simulink model "DC_MOTOR11"  (R2018a)
settings: Solver=FixedStepAuto  StartTime=0.0  StopTime=8  FixedStep=0.00001  RelTol=1e-3
values from neighbouring files (symbols this model uses):
  Bm = 0.0006    [dc1.m]
  Jm = 0.00233    [dc1.m]
  Kmm = 1    [dc1.m]
  Lam = 0.0017    [dc1.m]
  Lfm = 0.08    [dc1.m]
  Ram = 0.33    [dc1.m]
  Rfm = 3.33,    [dc1.m]
settings Model: ModifiedByFormat=LENOVO  Creator=Petar  LastModifiedBy=LENOVO

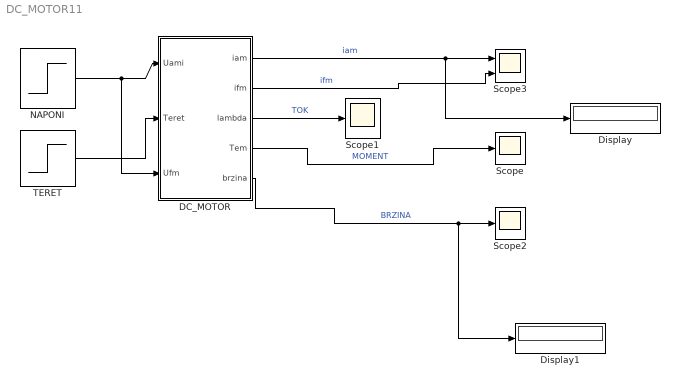
== system DC_MOTOR11 ==
  DC_MOTOR : Subsystem
  Display : Display
  Display1 : Display
  NAPONI : Step  After=24  SampleTime=0
  Scope : Scope
  Scope1 : Scope
  Scope2 : Scope
  Scope3 : Scope  NumInputPorts=2
  TERET : Step  After=27  SampleTime=0
  wires:
  NAPONI/1 -> DC_MOTOR/3(Ufm), DC_MOTOR/1("\tUami")
  TERET/1 -> DC_MOTOR/2(Teret)
  DC_MOTOR/1(iam) -> Display/1, Scope3/1  "iam"
  DC_MOTOR/2(ifm) -> Scope3/2  "ifm"
  DC_MOTOR/3(lambda) -> Scope1/1  "TOK"
  DC_MOTOR/4(Tem) -> Scope/1  "MOMENT"
  DC_MOTOR/5(brzina) -> Display1/1, Scope2/1  "BRZINA"

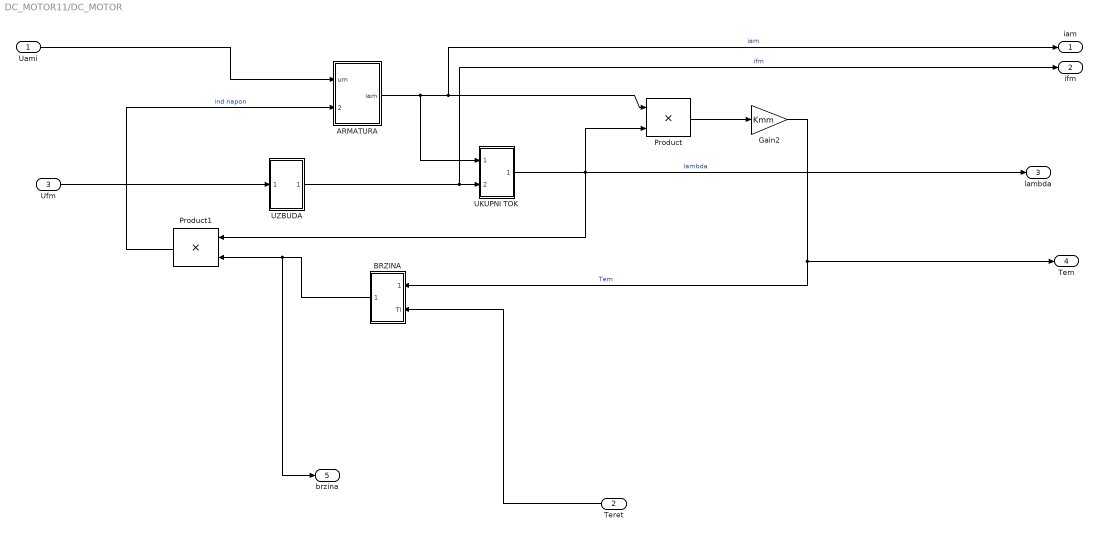
== system DC_MOTOR11/DC_MOTOR ==
  "\tUami" : Inport
  Teret : Inport  Port=2
  Ufm : Inport  Port=3
  ARMATURA : Subsystem
  BRZINA : Subsystem
  Gain2 : Gain  Gain=Kmm
  Product : Product
  Product1 : Product
  UKUPNI TOK : Subsystem
  UZBUDA : Subsystem
  iam : Outport
  ifm : Outport  Port=2
  lambda : Outport  Port=3
  Tem : Outport  Port=4
  brzina : Outport  Port=5
  wires:
  Gain2/1 -> Tem/1, BRZINA/1(Tem)  "Tem"
  UZBUDA/1(ifm) -> ifm/1, UKUPNI TOK/2(ifm)  "ifm"
  Teret/1 -> BRZINA/2(Tl)
  ARMATURA/1(iam) -> UKUPNI TOK/1(iam), iam/1, Product/1  "iam"
  BRZINA/1(wm) -> brzina/1, Product1/2
  Product1/1 -> ARMATURA/2(ind napon)  "ind napon"
  "\tUami"/1 -> ARMATURA/1(um)
  Product/1 -> Gain2/1
  UKUPNI TOK/1(lambda) -> lambda/1, Product1/1, Product/2  "lambda"
  Ufm/1 -> UZBUDA/1(Ufm)

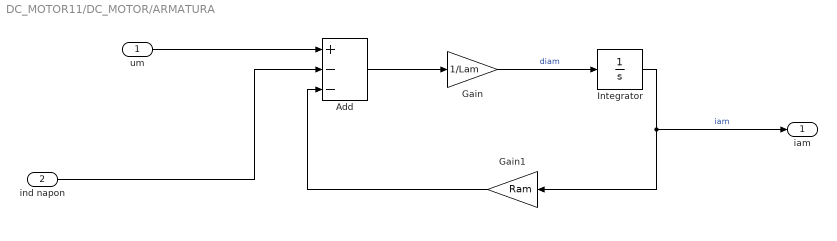
== system DC_MOTOR11/DC_MOTOR/ARMATURA ==
  um : Inport
  ind napon : Inport  Port=2
  Add : Sum  Inputs=+--
  Gain : Gain  Gain=1/Lam
  Gain1 : Gain  Gain=Ram
  Integrator : Integrator
  iam : Outport
  wires:
  Integrator/1 -> iam/1, Gain1/1  "iam"
  Gain/1 -> Integrator/1  "diam"
  Gain1/1 -> Add/3
  um/1 -> Add/1
  Add/1 -> Gain/1
  ind napon/1 -> Add/2

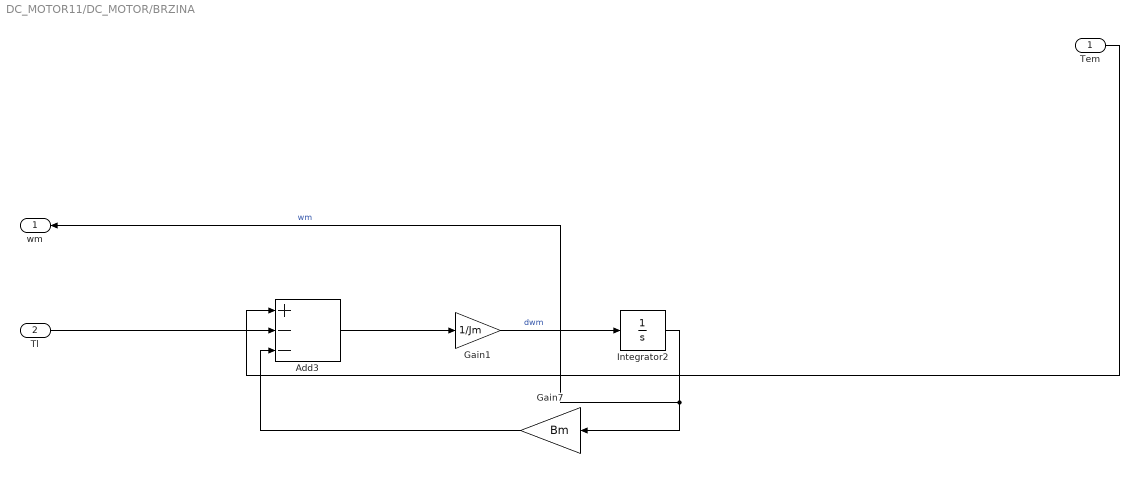
== system DC_MOTOR11/DC_MOTOR/BRZINA ==
  Tem : Inport
  Tl : Inport  Port=2
  Add3 : Sum  Inputs=+--
  Gain1 : Gain  Gain=1/Jm
  Gain7 : Gain  Gain=Bm
  Integrator2 : Integrator
  wm : Outport
  wires:
  Gain1/1 -> Integrator2/1  "dwm"
  Tl/1 -> Add3/2
  Gain7/1 -> Add3/3
  Integrator2/1 -> wm/1, Gain7/1  "wm"
  Add3/1 -> Gain1/1
  Tem/1 -> Add3/1

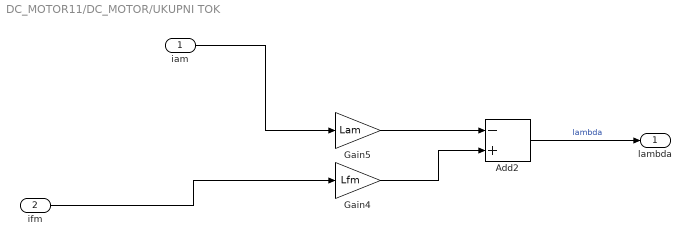
== system DC_MOTOR11/DC_MOTOR/UKUPNI TOK ==
  iam : Inport
  ifm : Inport  Port=2
  Add2 : Sum  Inputs=-+
  Gain4 : Gain  Gain=Lfm
  Gain5 : Gain  Gain=Lam
  lambda : Outport
  wires:
  Gain4/1 -> Add2/2
  Gain5/1 -> Add2/1
  iam/1 -> Gain5/1
  Add2/1 -> lambda/1  "lambda"
  ifm/1 -> Gain4/1

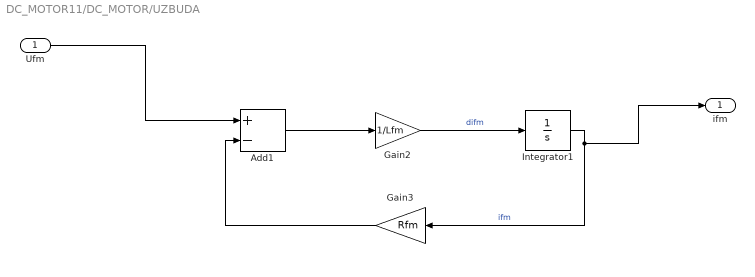
== system DC_MOTOR11/DC_MOTOR/UZBUDA ==
  Ufm : Inport
  Add1 : Sum  Inputs=+-
  Gain2 : Gain  Gain=1/Lfm
  Gain3 : Gain  Gain=Rfm
  Integrator1 : Integrator
  ifm : Outport
  wires:
  Integrator1/1 -> ifm/1, Gain3/1  "ifm"
  Add1/1 -> Gain2/1
  Gain2/1 -> Integrator1/1  "difm"
  Gain3/1 -> Add1/2
  Ufm/1 -> Add1/1
